simulink model "LQR_model"  (R2022a)
settings: Solver=VariableStepAuto  StartTime=0.0  StopTime=10.0  RelTol=1e-3
values from neighbouring files (symbols this model uses):
  A = 1    [LQR_Test_1D.m]    (also in LQR_Test_tracking_Delta_U_AD_MSD.m = sys_d.a; System_discretization.m = [0 1 0 0; discret_sys_calc.m = [0 1;-2 -3]; untitled.m = [0 1;-2 -3])
  B = 1    [LQR_Test_1D.m]    (also in LQR_Test_tracking_Delta_U_AD_MSD.m = sys_d.b; System_discretization.m = [0; discret_sys_calc.m = [0;1]; untitled.m = [0;1])
undefined symbols (not defined in the file or in its folder): BD, K, L
settings Model: Creator=罗恩泽  LastModifiedBy=Administrator
settings ModelReferenceCC: EnableRefExpFcnMdlSchedulingChecks=off
settings RTWCC: Description=Generic Real-Time Target

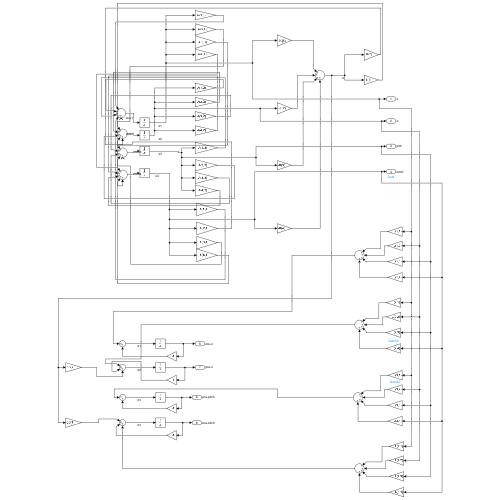
[thumbnail: Simulink's stored preview of the top-level diagram]
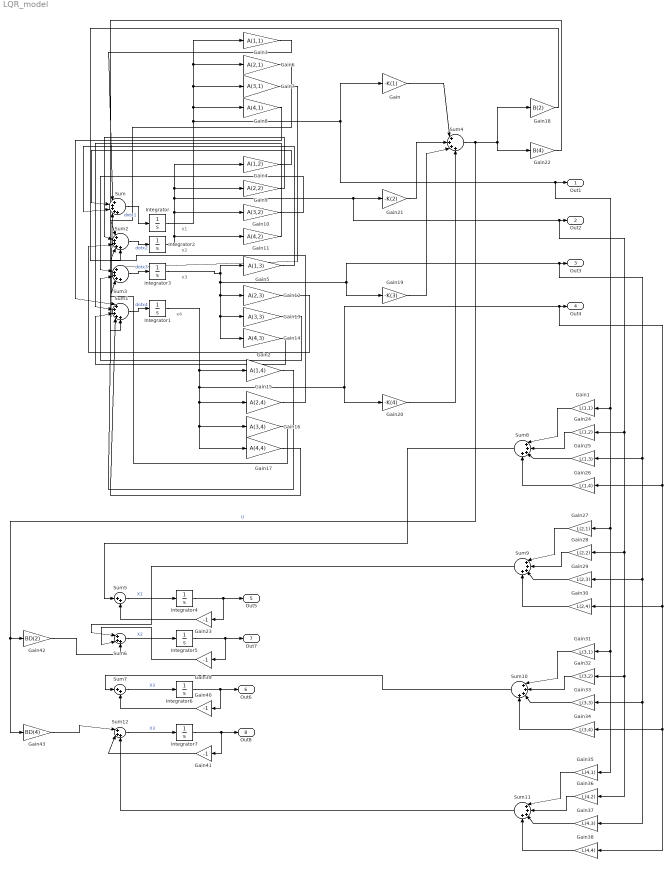
== system LQR_model ==
  note: x4
  note: x1
  note: x2
  note: x3
  Gain : Gain  Gain=-K(1)
  Gain1 : Gain  Gain=L(1,1)
  Gain10 : Gain  Gain=A(3,2)
  Gain11 : Gain  Gain=A(4,2)
  Gain12 : Gain  Gain=A(2,3)
  Gain13 : Gain  Gain=A(3,3)
  Gain14 : Gain  Gain=A(4,3)
  Gain15 : Gain  Gain=A(2,4)
  Gain16 : Gain  Gain=A(3,4)
  Gain17 : Gain  Gain=A(4,4)
  Gain18 : Gain  Gain=B(2)
  Gain19 : Gain  Gain=-K(3)
  Gain2 : Gain  Gain=A(1,4)
  Gain20 : Gain  Gain=-K(4)
  Gain21 : Gain  Gain=-K(2)
  Gain22 : Gain  Gain=B(4)
  Gain{23,39..41} (4 alike) : Gain  Gain=-1
  Gain24 : Gain  Gain=L(1,2)
  Gain25 : Gain  Gain=L(1,3)
  Gain26 : Gain  Gain=L(1,4)
  Gain27 : Gain  Gain=L(2,1)
  Gain28 : Gain  Gain=L(2,2)
  Gain29 : Gain  Gain=L(2,3)
  Gain3 : Gain  Gain=A(1,1)
  Gain30 : Gain  Gain=L(2,4)
  Gain31 : Gain  Gain=L(3,1)
  Gain32 : Gain  Gain=L(3,2)
  Gain33 : Gain  Gain=L(3,3)
  Gain34 : Gain  Gain=L(3,4)
  Gain35 : Gain  Gain=L(4,1)
  Gain36 : Gain  Gain=L(4,2)
  Gain37 : Gain  Gain=L(4,3)
  Gain38 : Gain  Gain=L(4,4)
  Gain4 : Gain  Gain=A(1,2)
  Gain42 : Gain  Gain=BD(2)
  Gain43 : Gain  Gain=BD(4)
  Gain5 : Gain  Gain=A(1,3)
  Gain6 : Gain  Gain=A(2,1)
  Gain7 : Gain  Gain=A(3,1)
  Gain8 : Gain  Gain=A(4,1)
  Gain9 : Gain  Gain=A(2,2)
  Integrator{,1,4..7} (6 alike) : Integrator
  Integrator2 : Integrator  InitialCondition=0.2
  Integrator3 : Integrator  InitialCondition=0.43
  Sum{,1..3} (4 alike) : Sum  Inputs=|+++++
  Sum{4,8..11} (5 alike) : Sum  Inputs=|++++
  Sum12 : Sum  Inputs=|+++
  Sum5 : Sum  Inputs=|++
  Sum6 : Sum  Inputs=|+++
  Sum7 : Sum  Inputs=|++
  Out1 : Outport  SignalName=x
  Out2 : Outport  Port=2  SignalName=x'
  Out3 : Outport  Port=3  SignalName=pith
  Out4 : Outport  Port=4  SignalName=pitch'
  Out5 : Outport  Port=5  SignalName=pre-x
  Out6 : Outport  Port=6  SignalName=pre-pitch
  Out7 : Outport  Port=7  SignalName=pre-x'
  Out8 : Outport  Port=8  SignalName=pre-pitch'
  wires:
  Sum/1 -> Integrator/1  "dotx1"
  Sum1/1 -> Integrator1/1  "dotx4"
  Integrator1/1 -> Gain38/1, Gain34/1, Gain30/1, Gain26/1, Out4/1, Gain20/1, Gain15/1, Gain17/1, Gain16/1, Gain2/1
  Integrator2/1 -> Gain36/1, Gain32/1, Gain28/1, Gain24/1, Out2/1, Gain21/1, Gain4/1, Gain9/1, Gain10/1, Gain11/1
  Sum2/1 -> Integrator2/1  "dotx2"
  Sum3/1 -> Integrator3/1  "dotx3"
  Integrator3/1 -> Gain37/1, Gain33/1, Gain29/1, Gain25/1, Out3/1, Gain19/1, Gain14/1, Gain13/1, Gain12/1, Gain5/1
  Integrator/1 -> Gain35/1, Gain31/1, Gain27/1, Gain1/1, Out1/1, Gain/1, Gain3/1, Gain6/1, Gain7/1, Gain8/1
  Gain3/1 -> Sum/1
  Gain4/1 -> Sum/2
  Gain5/1 -> Sum/3
  Gain2/1 -> Sum/4
  Gain6/1 -> Sum2/1
  Gain8/1 -> Sum1/1
  Gain9/1 -> Sum2/2
  Gain7/1 -> Sum3/1
  Gain10/1 -> Sum3/2
  Gain11/1 -> Sum1/2
  Gain12/1 -> Sum2/3
  Gain13/1 -> Sum3/3
  Gain14/1 -> Sum1/3
  Gain15/1 -> Sum2/4
  Gain16/1 -> Sum3/4
  Gain17/1 -> Sum1/4
  Gain/1 -> Sum4/1
  Gain21/1 -> Sum4/2
  Gain19/1 -> Sum4/3
  Gain20/1 -> Sum4/4
  Sum4/1 -> Gain43/1, Gain42/1, Gain22/1, Gain18/1  "U"
  Gain22/1 -> Sum1/5
  Gain18/1 -> Sum2/5
  Sum5/1 -> Integrator4/1  "X1"
  Sum6/1 -> Integrator5/1  "X2"
  Integrator5/1 -> Gain39/1, Out7/1
  Sum7/1 -> Integrator6/1  "X3"
  Integrator6/1 -> Gain40/1, Out6/1
  Integrator4/1 -> Gain23/1, Out5/1
  Gain1/1 -> Sum8/1
  Gain24/1 -> Sum8/2
  Gain25/1 -> Sum8/3
  Gain26/1 -> Sum8/4
  Gain27/1 -> Sum9/1
  Gain28/1 -> Sum9/2
  Gain29/1 -> Sum9/3
  Gain30/1 -> Sum9/4
  Gain31/1 -> Sum10/1
  Gain32/1 -> Sum10/2
  Gain33/1 -> Sum10/3
  Gain34/1 -> Sum10/4
  Gain35/1 -> Sum11/1
  Gain36/1 -> Sum11/2
  Gain38/1 -> Sum11/4
  Gain37/1 -> Sum11/3
  Sum8/1 -> Sum5/1
  Integrator7/1 -> Gain41/1, Out8/1
  Sum12/1 -> Integrator7/1  "X3"
  Sum9/1 -> Sum6/1
  Sum10/1 -> Sum7/1
  Sum11/1 -> Sum12/3
  Gain23/1 -> Sum5/2
  Gain39/1 -> Sum6/2
  Gain40/1 -> Sum7/2
  Gain41/1 -> Sum12/2
  Gain42/1 -> Sum6/3
  Gain43/1 -> Sum12/1
